simulink model "trajTest"  (R2016b)
settings: Solver=VariableStepAuto  StartTime=0.0  StopTime=0.6  FixedStep=5e-5  RelTol=1e-3
libraries: model_controller x4
settings Model: Creator=Dai Luyao  LastModifiedBy=Dai Luyao

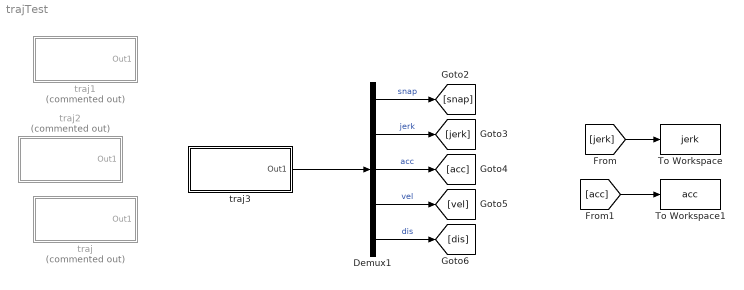
== system trajTest ==
  Demux1 : Demux  Outputs=5
  To Workspace : ToWorkspace  VariableName=jerk  SaveFormat=Structure With Time  SampleTime=-1
  To Workspace1 : ToWorkspace  VariableName=acc  SaveFormat=Structure With Time  SampleTime=-1
  traj : Subsystem  Commented=on  BlockChoice=4th order traj
      link override 4th order traj: v=0.5  x=0.1  j=500
      settings: AttributesFormatString=%<BlockChoice>  TemplateBlock=model_controller/Profile Generators/traj  MemberBlocks=2th order traj,3rd order traj,4th order traj,step
  traj1 : Subsystem  Commented=on  BlockChoice=4th order traj
      link override 4th order traj: v=0.25
      settings: AttributesFormatString=%<BlockChoice>  TemplateBlock=model_controller/Profile Generators/traj  MemberBlocks=2th order traj,3rd order traj,4th order traj,step
  traj2 : Subsystem  Commented=on  BlockChoice=4th order traj
      link override 4th order traj: v=0.6  x=0.1  j=700  d=20000
      settings: AttributesFormatString=%<BlockChoice>  TemplateBlock=model_controller/Profile Generators/traj  MemberBlocks=2th order traj,3rd order traj,4th order traj,step
  traj3 : Subsystem  BlockChoice=4th order traj
      link override 4th order traj: v=0.2  x=0.1  a=5
      settings: AttributesFormatString=%<BlockChoice>  TemplateBlock=model_controller/Profile Generators/traj  MemberBlocks=2th order traj,3rd order traj,4th order traj,step
  wires:
  Demux1/1 -> [snap]  "snap"
  Demux1/2 -> [jerk]  "jerk"
  Demux1/3 -> [acc]  "acc"
  Demux1/4 -> [vel]  "vel"
  Demux1/5 -> [dis]  "dis"
  [acc] -> To Workspace1/1
  [jerk] -> To Workspace/1
  traj3/1(Out1) -> Demux1/1

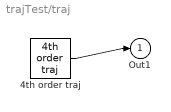
== system trajTest/traj ==
  4th order traj : model_controller/Profile Generators/4th order traj  t0=0  x=0.1  v=0.5  a=10  j=500  d=64000  Ts=0
  Out1 : Outport
  wires:
  4th order traj/1 -> Out1/1

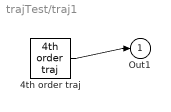
== system trajTest/traj1 ==
  4th order traj : model_controller/Profile Generators/4th order traj  t0=0  x=0.06  v=0.25  a=10  j=800  d=64000  Ts=0
  Out1 : Outport
  wires:
  4th order traj/1 -> Out1/1

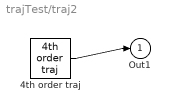
== system trajTest/traj2 ==
  4th order traj : model_controller/Profile Generators/4th order traj  t0=0  x=0.1  v=0.6  a=10  j=700  d=20000  Ts=0
  Out1 : Outport
  wires:
  4th order traj/1 -> Out1/1

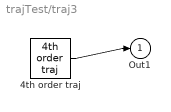
== system trajTest/traj3 ==
  4th order traj : model_controller/Profile Generators/4th order traj  t0=0  x=0.1  v=0.2  a=5  j=800  d=64000  Ts=0
  Out1 : Outport
  wires:
  4th order traj/1 -> Out1/1
